simulink library "thc"  (R2021b)
settings: Solver=VariableStepAuto  StartTime=0.0  StopTime=10.0  RelTol=1e-3
undefined symbols (not defined in the file or in its folder): ATHC_APTCQA_X_C, ATHC_APTCQB_X_C, ATHC_dAy_X_C, ATHC_Qeq_X_kmh, ATHC_VbaseC_X_C, ATHC_VbaseC_Y_W, ATHC_VbaseD_X_C, ATHC_VbaseH_X_C, FALSE, KTHC_ACMaxMinT_sec, KTHC_aDeice_K, KTHC_AGSDefLv_K, KTHC_AGSLv1_K, KTHC_AGSLv2_K, KTHC_AGSLv3_K, KTHC_AGSLv4_K, KTHC_AGSLv5_K, KTHC_AirIntUpdateT_sec, KTHC_APTCOneZoneMax_W, KTHC_APTCQMaxC_W, KTHC_APTCQminC_W, KTHC_APTCQminD_W, KTHC_APTCQminRe1_W, KTHC_APTCQminRe_W, KTHC_APTCQoffT_cnt, KTHC_APTCQonT_cnt, KTHC_APTCRiLeMaxDff_W, KTHC_APTCRiLeMinDff_W, KTHC_BatInTempDef_C, KTHC_bDeice_K, KTHC_CompMaxDeice_rpm, KTHC_CompMinDeice_rpm, KTHC_CompSotxvOp_K, KTHC_CompSotxvOpLow_rpm, KTHC_CompSpdmax_rpm, KTHC_CompSpdmaxBC1_rpm, KTHC_CompSpdmaxBC_rpm, KTHC_CompSpdmid1_rpm, KTHC_CompSpdmid2_rpm, KTHC_CompSpdmid3_rpm, KTHC_CompSpdmid_rpm, KTHC_CompSpdmin_rpm, KTHC_DAPTCQ1_W, KTHC_DAPTCQ2_W, KTHC_DAPTCQ3_W, KTHC_DcChSetTemp_C, KTHC_DehumidityEN_flg, KTHC_DeiceCycTime_K, KTHC_DTambSat1_C, KTHC_DTambSat2_C, KTHC_DTambsat3_C, KTHC_DTambsat4_C, KTHC_DTambSat5_C, KTHC_DTambSat_C, KTHC_DTcabin10_C, KTHC_DTCabin11_C, KTHC_DTcabin12_C, KTHC_DTcabin1_C, KTHC_DTcabin2_C, KTHC_DTcabin3_C ... (+347)
libraries: simulink x80
(part 8 of 8)

== stateflow chart thc/THC/ThermalControl/THCM_Conctrl/Subsystem/Chart ==
  state ForceCompOFF
    en:FCompOFF=True;
    Keep=True;
    EXVOpen=1;
  state StandBy
    en:FCompOFF=False;
    Keep=False;
    EXVOpen=0;
  state ForceCompOFF3
    en:
    Keep=False;
    EXVOpen=0;
  note: 2 sec
  note: 5 sec
  note: 5 sec
  state ForceCompOFF2
    en:
    Keep=False;
    EXVOpen=0;
  state ForceCompOFF1
    en:
    Keep=True;
    EXVOpen=2;
  note: 10 sec
  (default) -> StandBy
  StandBy -> (junction 26) : [SOV1C!=SOV1CBuf||SOV2C!=SOV2CBuf||SOV3C!=SOV3CBuf]
  (junction 26) -> ForceCompOFF [order 2]
  (junction 26) -> ForceCompOFF3 [order 1] : [Comp==0]{FCompOFF=True;}
  ForceCompOFF -> ForceCompOFF1 : [after(KTHC_PBlaceTime1_K,tick)]
  ForceCompOFF3 -> StandBy : [after(KTHC_PBlaceTime4_K,tick)]
  ForceCompOFF2 -> StandBy : [after(KTHC_PBlaceTime3_K,tick)]
  ForceCompOFF1 -> ForceCompOFF2 : [after(KTHC_PBlaceTime2_K,tick)]
  data: FCompOFF output boolean; SOV1C input; SOV1CBuf input; SOV2C input; SOV2CBuf input; SOV3C input; SOV3CBuf input; Keep output boolean; True constant boolean =boolean(1); False constant boolean =boolean(0); Comp input; KTHC_PBlaceTime1_K input; KTHC_PBlaceTime2_K input; KTHC_PBlaceTime3_K input; KTHC_PBlaceTime4_K input; EXVOpenflg local boolean; EXVOpen output uint8
